simulink model "Three_Phase_Templates"  (R2021a)
settings: Solver=VariableStepAuto  StartTime=0.0  StopTime=10.0  RelTol=1e-3
libraries: fl_lib x35, nesl_utility x22, ee_lib x7, spsFourierLib x3, simulink_extras x1
settings Model: Creator=bemen  LastModifiedBy=bemen

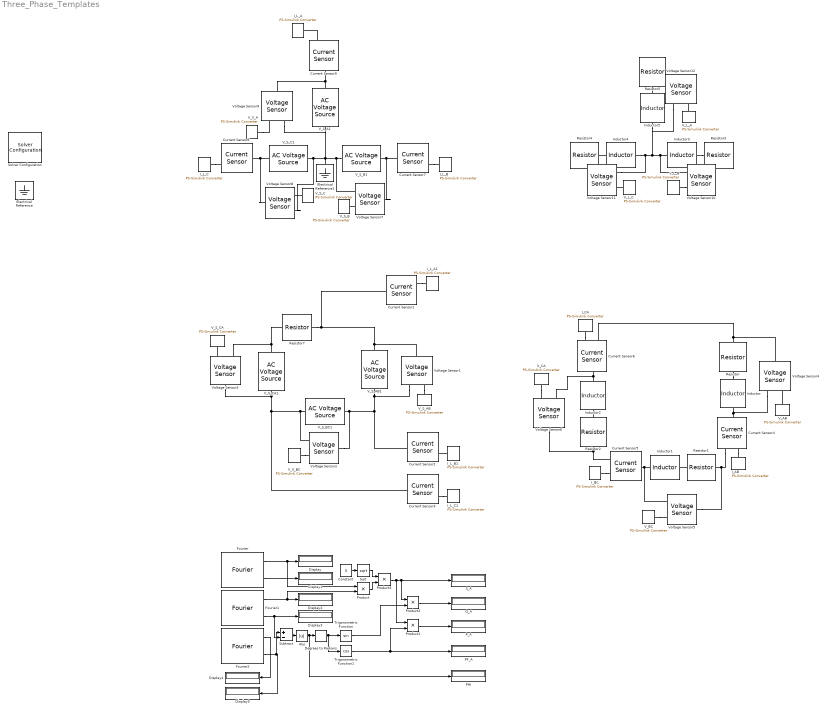
== system Three_Phase_Templates ==
  Abs : Abs
  Constant : Constant  Value=3
  Current Sensor{1..9} (9 alike) : fl_lib/Electrical/Electrical Sensors/Current Sensor
  Degrees to Radians : simulink_extras/Transformations/Degrees to Radians
  Display{,1..5} (6 alike) : Display
  Electrical Reference : fl_lib/Electrical/Electrical Elements/Electrical Reference
  Electrical Reference1 : fl_lib/Electrical/Electrical Elements/Electrical Reference
  Fourier : spsFourierLib/Fourier  Freq=60  n=1  InInit=[0, 0]  Ts=0
      settings: SourceProductBaseCode=PS
  Fourier1 : spsFourierLib/Fourier  Freq=60  n=1  InInit=[0, 0]  Ts=0
      settings: SourceProductBaseCode=PS
  Fourier2 : spsFourierLib/Fourier  Freq=60  n=1  InInit=[0, 0]  Ts=0
      settings: SourceProductBaseCode=PS
  I_AB : nesl_utility/PS-Simulink Converter  PhysicalDomain=network_engine_domain  SubClassName=ps_output  LeftPortType=input  RightPortType=output  PseudoPeriodic=off  Frequencies=[]  Unit=inherit  AffineConversion=off
      settings: SourceProductBaseCode=PW,SS
  I_BC : nesl_utility/PS-Simulink Converter  PhysicalDomain=network_engine_domain  SubClassName=ps_output  LeftPortType=input  RightPortType=output  PseudoPeriodic=off  Frequencies=[]  Unit=inherit  AffineConversion=off
      settings: SourceProductBaseCode=PW,SS
  I_CA : nesl_utility/PS-Simulink Converter  PhysicalDomain=network_engine_domain  SubClassName=ps_output  LeftPortType=input  RightPortType=output  PseudoPeriodic=off  Frequencies=[]  Unit=inherit  AffineConversion=off
      settings: SourceProductBaseCode=PW,SS
  I_L_A : nesl_utility/PS-Simulink Converter  PhysicalDomain=network_engine_domain  SubClassName=ps_output  LeftPortType=input  RightPortType=output  PseudoPeriodic=off  Frequencies=[]  Unit=inherit  AffineConversion=off
      settings: SourceProductBaseCode=PW,SS
  I_L_A1 : nesl_utility/PS-Simulink Converter  PhysicalDomain=network_engine_domain  SubClassName=ps_output  LeftPortType=input  RightPortType=output  PseudoPeriodic=off  Frequencies=[]  Unit=inherit  AffineConversion=off
      settings: SourceProductBaseCode=PW,SS
  I_L_B : nesl_utility/PS-Simulink Converter  PhysicalDomain=network_engine_domain  SubClassName=ps_output  LeftPortType=input  RightPortType=output  PseudoPeriodic=off  Frequencies=[]  Unit=inherit  AffineConversion=off
      settings: SourceProductBaseCode=PW,SS
  I_L_B1 : nesl_utility/PS-Simulink Converter  PhysicalDomain=network_engine_domain  SubClassName=ps_output  LeftPortType=input  RightPortType=output  PseudoPeriodic=off  Frequencies=[]  Unit=inherit  AffineConversion=off
      settings: SourceProductBaseCode=PW,SS
  I_L_C : nesl_utility/PS-Simulink Converter  PhysicalDomain=network_engine_domain  SubClassName=ps_output  LeftPortType=input  RightPortType=output  PseudoPeriodic=off  Frequencies=[]  Unit=inherit  AffineConversion=off
      settings: SourceProductBaseCode=PW,SS
  I_L_C1 : nesl_utility/PS-Simulink Converter  PhysicalDomain=network_engine_domain  SubClassName=ps_output  LeftPortType=input  RightPortType=output  PseudoPeriodic=off  Frequencies=[]  Unit=inherit  AffineConversion=off
      settings: SourceProductBaseCode=PW,SS
  Inductor{,1..5} (6 alike) : fl_lib/Electrical/Electrical Elements/Inductor  l=13.26291192 mH  r=0 Ohm  g=1e-9 1/Ohm  i_specify=off  i_priority=None  i=0 A  i_nominal_specify=off  i_nominal_unit=A  i_nominal_value=1  v_specify=off  v_priority=None  v=0 V  v_nominal_specify=off  v_nominal_unit=V  v_nominal_value=1  i_L_specify=off  i_L_priority=High  i_L=0 A  i_L_nominal_specify=off  i_L_nominal_unit=A  i_L_nominal_value=1
  PF_A : Display
  PHI : Display
  P_A : Display
  Product{,1..3} (4 alike) : Product
  Q_A : Display
  Resistor : ee_lib/Passive/Resistor  R=5 Ohm  R_tol=5  enable_R_tol=0  tol_distribution=1  nSigma=4  enable_operating_limits=0  operating_limit_action=2  max_working_voltage=100 V  power_rating=1 W  enable_faults=0  fault_action=1  R_faulted=inf Ohm  enable_temporal_fault=0  t_fault=1 s  enable_behavioral_fault=0  max_permissible_current=1 A  t_fail_on_current=1 s  noise_mode=0  sample_time=1e-3 s  repeatability=1  auto_seed=19903842  user_seed=0  Tdevice=25 degC  alpha=3.93e-3 1/K  Tmeas=25 degC  thermal_mass=100 J/K  power_derating_T1=70 degC  power_derating_T2=155 degC  operating_temperature_range_vec=[-50, 150] degC  temperature_specify=off  temperature_priority=High  temperature=298.15 K  temperature_nominal_specify=off  temperature_nominal_unit=K  temperature_nominal_value=1
  Resistor1 : ee_lib/Passive/Resistor  R=5 Ohm  R_tol=5  enable_R_tol=0  tol_distribution=1  nSigma=4  enable_operating_limits=0  operating_limit_action=2  max_working_voltage=100 V  power_rating=1 W  enable_faults=0  fault_action=1  R_faulted=inf Ohm  enable_temporal_fault=0  t_fault=1 s  enable_behavioral_fault=0  max_permissible_current=1 A  t_fail_on_current=1 s  noise_mode=0  sample_time=1e-3 s  repeatability=1  auto_seed=3510290603  user_seed=0  Tdevice=25 degC  alpha=3.93e-3 1/K  Tmeas=25 degC  thermal_mass=100 J/K  power_derating_T1=70 degC  power_derating_T2=155 degC  operating_temperature_range_vec=[-50, 150] degC  temperature_specify=off  temperature_priority=High  temperature=298.15 K  temperature_nominal_specify=off  temperature_nominal_unit=K  temperature_nominal_value=1
  Resistor2 : ee_lib/Passive/Resistor  R=5 Ohm  R_tol=5  enable_R_tol=0  tol_distribution=1  nSigma=4  enable_operating_limits=0  operating_limit_action=2  max_working_voltage=100 V  power_rating=1 W  enable_faults=0  fault_action=1  R_faulted=inf Ohm  enable_temporal_fault=0  t_fault=1 s  enable_behavioral_fault=0  max_permissible_current=1 A  t_fail_on_current=1 s  noise_mode=0  sample_time=1e-3 s  repeatability=1  auto_seed=3731015349  user_seed=0  Tdevice=25 degC  alpha=3.93e-3 1/K  Tmeas=25 degC  thermal_mass=100 J/K  power_derating_T1=70 degC  power_derating_T2=155 degC  operating_temperature_range_vec=[-50, 150] degC  temperature_specify=off  temperature_priority=High  temperature=298.15 K  temperature_nominal_specify=off  temperature_nominal_unit=K  temperature_nominal_value=1
  Resistor3 : ee_lib/Passive/Resistor  R=5 Ohm  R_tol=5  enable_R_tol=0  tol_distribution=1  nSigma=4  enable_operating_limits=0  operating_limit_action=2  max_working_voltage=100 V  power_rating=1 W  enable_faults=0  fault_action=1  R_faulted=inf Ohm  enable_temporal_fault=0  t_fault=1 s  enable_behavioral_fault=0  max_permissible_current=1 A  t_fail_on_current=1 s  noise_mode=0  sample_time=1e-3 s  repeatability=1  auto_seed=362649195  user_seed=0  Tdevice=25 degC  alpha=3.93e-3 1/K  Tmeas=25 degC  thermal_mass=100 J/K  power_derating_T1=70 degC  power_derating_T2=155 degC  operating_temperature_range_vec=[-50, 150] degC  temperature_specify=off  temperature_priority=High  temperature=298.15 K  temperature_nominal_specify=off  temperature_nominal_unit=K  temperature_nominal_value=1
  Resistor4 : ee_lib/Passive/Resistor  R=5 Ohm  R_tol=5  enable_R_tol=0  tol_distribution=1  nSigma=4  enable_operating_limits=0  operating_limit_action=2  max_working_voltage=100 V  power_rating=1 W  enable_faults=0  fault_action=1  R_faulted=inf Ohm  enable_temporal_fault=0  t_fault=1 s  enable_behavioral_fault=0  max_permissible_current=1 A  t_fail_on_current=1 s  noise_mode=0  sample_time=1e-3 s  repeatability=1  auto_seed=1717053403  user_seed=0  Tdevice=25 degC  alpha=3.93e-3 1/K  Tmeas=25 degC  thermal_mass=100 J/K  power_derating_T1=70 degC  power_derating_T2=155 degC  operating_temperature_range_vec=[-50, 150] degC  temperature_specify=off  temperature_priority=High  temperature=298.15 K  temperature_nominal_specify=off  temperature_nominal_unit=K  temperature_nominal_value=1
  Resistor5 : ee_lib/Passive/Resistor  R=5 Ohm  R_tol=5  enable_R_tol=0  tol_distribution=1  nSigma=4  enable_operating_limits=0  operating_limit_action=2  max_working_voltage=100 V  power_rating=1 W  enable_faults=0  fault_action=1  R_faulted=inf Ohm  enable_temporal_fault=0  t_fault=1 s  enable_behavioral_fault=0  max_permissible_current=1 A  t_fail_on_current=1 s  noise_mode=0  sample_time=1e-3 s  repeatability=1  auto_seed=1116134882  user_seed=0  Tdevice=25 degC  alpha=3.93e-3 1/K  Tmeas=25 degC  thermal_mass=100 J/K  power_derating_T1=70 degC  power_derating_T2=155 degC  operating_temperature_range_vec=[-50, 150] degC  temperature_specify=off  temperature_priority=High  temperature=298.15 K  temperature_nominal_specify=off  temperature_nominal_unit=K  temperature_nominal_value=1
  Resistor7 : ee_lib/Passive/Resistor  R=0.000001 Ohm  R_tol=5  enable_R_tol=0  tol_distribution=1  nSigma=4  enable_operating_limits=0  operating_limit_action=2  max_working_voltage=100 V  power_rating=1 W  enable_faults=0  fault_action=1  R_faulted=inf Ohm  enable_temporal_fault=0  t_fault=1 s  enable_behavioral_fault=0  max_permissible_current=1 A  t_fail_on_current=1 s  noise_mode=0  sample_time=1e-3 s  repeatability=1  auto_seed=189689687  user_seed=0  Tdevice=25 degC  alpha=3.93e-3 1/K  Tmeas=25 degC  thermal_mass=100 J/K  power_derating_T1=70 degC  power_derating_T2=155 degC  operating_temperature_range_vec=[-50, 150] degC  temperature_specify=off  temperature_priority=High  temperature=298.15 K  temperature_nominal_specify=off  temperature_nominal_unit=K  temperature_nominal_value=1
  S_A : Display
  Solver Configuration : nesl_utility/Solver Configuration  PhysicalDomain=network_engine_domain  SubClassName=solver  LeftPortType=input  RightPortType=generic  Tones=[]  Harmonics=[]  SimulateNoise=off  Profile=off  UseLocalSampling=off  EnableSwitchedLinearOptims=on  FrequencyDomain=off  UseCCode=off  RelTol=0.001  AbsTol=1e-06  MinStep=1e-09  ToWorkspace=off  RevertToSquareIcSolve=off  NumHomotopyIterations=100  PhasorMode=off  PhasorModeNumHarmonics=1  DoDC=on  ResidualTolerance=1e-09  UseLocalSolver=off  LocalSolverChoice=NE_BACKWARD_EULER_ADVANCER  LocalSolverSampleTime=0.001  DoFixedCost=off  MaxNonlinIter=3  MaxModeIter=2  ComputeImpulses=off  ImpulseIterations=2  LinearAlgebra=auto  EquationFormulation=NE_TIME_EF  DelaysMemoryBudget=1024  AutomaticFiltering=on  FilteringTimeConstant=0.001  PartitionStorageMethod=AS_NEEDED  PartitionMemoryBudget=1024  PartitionMethod=ROBUST
      settings: SourceProductBaseCode=PW,SS
  Sqrt : Sqrt  SaturateOnIntegerOverflow=on
  Subtract : Sum  Inputs=+-
  Trigonometric Function : Trigonometry
  Trigonometric Function1 : Trigonometry  Operator=cos
  V_AB : nesl_utility/PS-Simulink Converter  PhysicalDomain=network_engine_domain  SubClassName=ps_output  LeftPortType=input  RightPortType=output  PseudoPeriodic=off  Frequencies=[]  Unit=inherit  AffineConversion=off
      settings: SourceProductBaseCode=PW,SS
  V_BC : nesl_utility/PS-Simulink Converter  PhysicalDomain=network_engine_domain  SubClassName=ps_output  LeftPortType=input  RightPortType=output  PseudoPeriodic=off  Frequencies=[]  Unit=inherit  AffineConversion=off
      settings: SourceProductBaseCode=PW,SS
  V_CA : nesl_utility/PS-Simulink Converter  PhysicalDomain=network_engine_domain  SubClassName=ps_output  LeftPortType=input  RightPortType=output  PseudoPeriodic=off  Frequencies=[]  Unit=inherit  AffineConversion=off
      settings: SourceProductBaseCode=PW,SS
  V_L_A : nesl_utility/PS-Simulink Converter  PhysicalDomain=network_engine_domain  SubClassName=ps_output  LeftPortType=input  RightPortType=output  PseudoPeriodic=off  Frequencies=[]  Unit=inherit  AffineConversion=off
      settings: SourceProductBaseCode=PW,SS
  V_L_B : nesl_utility/PS-Simulink Converter  PhysicalDomain=network_engine_domain  SubClassName=ps_output  LeftPortType=input  RightPortType=output  PseudoPeriodic=off  Frequencies=[]  Unit=inherit  AffineConversion=off
      settings: SourceProductBaseCode=PW,SS
  V_L_C : nesl_utility/PS-Simulink Converter  PhysicalDomain=network_engine_domain  SubClassName=ps_output  LeftPortType=input  RightPortType=output  PseudoPeriodic=off  Frequencies=[]  Unit=inherit  AffineConversion=off
      settings: SourceProductBaseCode=PW,SS
  V_S_A : nesl_utility/PS-Simulink Converter  PhysicalDomain=network_engine_domain  SubClassName=ps_output  LeftPortType=input  RightPortType=output  PseudoPeriodic=off  Frequencies=[]  Unit=inherit  AffineConversion=off
      settings: SourceProductBaseCode=PW,SS
  V_S_A1 : fl_lib/Electrical/Electrical Sources/AC Voltage Source  amp=120 V  shift=0 deg  frequency=60 Hz  omega=0 rad/s
  V_S_AB : nesl_utility/PS-Simulink Converter  PhysicalDomain=network_engine_domain  SubClassName=ps_output  LeftPortType=input  RightPortType=output  PseudoPeriodic=off  Frequencies=[]  Unit=inherit  AffineConversion=off
      settings: SourceProductBaseCode=PW,SS
  V_S_AB1 : fl_lib/Electrical/Electrical Sources/AC Voltage Source  amp=120 V  shift=0 deg  frequency=60 Hz  omega=0 rad/s
  V_S_B : nesl_utility/PS-Simulink Converter  PhysicalDomain=network_engine_domain  SubClassName=ps_output  LeftPortType=input  RightPortType=output  PseudoPeriodic=off  Frequencies=[]  Unit=inherit  AffineConversion=off
      settings: SourceProductBaseCode=PW,SS
  V_S_B1 : fl_lib/Electrical/Electrical Sources/AC Voltage Source  amp=120 V  shift=-120 deg  frequency=60 Hz  omega=0 rad/s
  V_S_BC : nesl_utility/PS-Simulink Converter  PhysicalDomain=network_engine_domain  SubClassName=ps_output  LeftPortType=input  RightPortType=output  PseudoPeriodic=off  Frequencies=[]  Unit=inherit  AffineConversion=off
      settings: SourceProductBaseCode=PW,SS
  V_S_BC1 : fl_lib/Electrical/Electrical Sources/AC Voltage Source  amp=120 V  shift=-120 deg  frequency=60 Hz  omega=0 rad/s
  V_S_C : nesl_utility/PS-Simulink Converter  PhysicalDomain=network_engine_domain  SubClassName=ps_output  LeftPortType=input  RightPortType=output  PseudoPeriodic=off  Frequencies=[]  Unit=inherit  AffineConversion=off
      settings: SourceProductBaseCode=PW,SS
  V_S_C1 : fl_lib/Electrical/Electrical Sources/AC Voltage Source  amp=120 V  shift=120 deg  frequency=60 Hz  omega=0 rad/s
  V_S_CA : nesl_utility/PS-Simulink Converter  PhysicalDomain=network_engine_domain  SubClassName=ps_output  LeftPortType=input  RightPortType=output  PseudoPeriodic=off  Frequencies=[]  Unit=inherit  AffineConversion=off
      settings: SourceProductBaseCode=PW,SS
  V_S_CA1 : fl_lib/Electrical/Electrical Sources/AC Voltage Source  amp=120 V  shift=120 deg  frequency=60 Hz  omega=0 rad/s
  Voltage Sensor{1..12} (12 alike) : fl_lib/Electrical/Electrical Sensors/Voltage Sensor
  wires:
  Fourier2/1 -> Display4/1
  Product3/1 -> Product1/1, Product2/1, S_A/1
  Product/1 -> Product3/2
  Fourier1/1 -> Product/2, Display2/1
  Abs/1 -> PHI/1, Degrees to Radians/1
  Product1/1 -> P_A/1
  Fourier/1 -> Product/1, Display/1
  Constant/1 -> Sqrt/1
  Sqrt/1 -> Product3/1
  Product2/1 -> Q_A/1
  Fourier/2 -> Display1/1
  Degrees to Radians/1 -> Trigonometric Function1/1, Trigonometric Function/1
  Trigonometric Function/1 -> Product2/2
  Trigonometric Function1/1 -> Product1/2, PF_A/1
  Fourier1/2 -> Subtract/2, Display3/1
  Fourier2/2 -> Subtract/1, Display5/1
  Subtract/1 -> Abs/1
  connections:
  V_S_AB1/RConn1 -- Voltage Sensor1/RConn2 -- Current Sensor2/LConn1 -- Voltage Sensor2/LConn1 -- V_S_BC1/LConn1
  V_S_BC1/RConn1 -- Voltage Sensor2/RConn2 -- Voltage Sensor3/LConn1 -- V_S_CA1/LConn1 -- Current Sensor3/LConn1
  Voltage Sensor3/RConn2 -- V_S_CA1/RConn1 -- Resistor7/LConn1
  Inductor/RConn1 -- Current Sensor4/LConn1 -- Voltage Sensor4/RConn2
  Resistor/RConn1 -- Inductor/LConn1
  Resistor1/RConn1 -- Inductor1/LConn1
  Resistor2/RConn1 -- Inductor2/LConn1
  Inductor2/RConn1 -- Voltage Sensor6/RConn2 -- Current Sensor6/LConn1
  Inductor1/RConn1 -- Voltage Sensor5/RConn2 -- Current Sensor5/LConn1
  Current Sensor6/RConn2 -- Voltage Sensor4/LConn1 -- Resistor/LConn1
  Resistor2/LConn1 -- Voltage Sensor6/LConn1 -- Current Sensor5/RConn2
  Current Sensor4/RConn2 -- Voltage Sensor5/LConn1 -- Resistor1/LConn1
  Current Sensor4/RConn1 -- I_AB/LConn1
  V_AB/LConn1 -- Voltage Sensor4/RConn1
  V_BC/LConn1 -- Voltage Sensor5/RConn1
  I_BC/LConn1 -- Current Sensor5/RConn1
  V_CA/LConn1 -- Voltage Sensor6/RConn1
  I_CA/LConn1 -- Current Sensor6/RConn1
  Voltage Sensor7/LConn1 -- Current Sensor7/LConn1 -- V_S_B1/LConn1
  V_S_C1/LConn1 -- Voltage Sensor8/LConn1 -- Current Sensor8/LConn1
  V_S_C1/RConn1 -- Voltage Sensor8/RConn2 -- Voltage Sensor9/RConn2 -- V_S_A1/RConn1 -- Electrical Reference1/LConn1 -- Voltage Sensor7/RConn2 -- V_S_B1/RConn1
  V_S_A1/LConn1 -- Voltage Sensor9/LConn1 -- Current Sensor9/LConn1
  Inductor3/LConn1 -- Resistor3/RConn1
  Inductor4/LConn1 -- Resistor4/RConn1
  Inductor5/LConn1 -- Resistor5/RConn1
  Inductor4/RConn1 -- Voltage Sensor11/RConn2 -- Voltage Sensor12/RConn2 -- Inductor5/RConn1 -- Voltage Sensor10/RConn2 -- Inductor3/RConn1
  V_L_B/LConn1 -- Voltage Sensor10/RConn1
  V_L_C/LConn1 -- Voltage Sensor11/RConn1
  V_L_A/LConn1 -- Voltage Sensor12/RConn1
  V_S_B/LConn1 -- Voltage Sensor7/RConn1
  V_S_C/LConn1 -- Voltage Sensor8/RConn1
  V_S_A/LConn1 -- Voltage Sensor9/RConn1
  Current Sensor7/RConn1 -- I_L_B/LConn1
  I_L_C/LConn1 -- Current Sensor8/RConn1
  Current Sensor9/RConn1 -- I_L_A/LConn1
  Voltage Sensor1/RConn1 -- V_S_AB/LConn1
  I_L_B1/LConn1 -- Current Sensor2/RConn1
  Current Sensor3/RConn1 -- I_L_C1/LConn1
  V_S_BC/LConn1 -- Voltage Sensor2/RConn1
  Voltage Sensor3/RConn1 -- V_S_CA/LConn1
  Current Sensor1/RConn1 -- I_L_A1/LConn1
  Current Sensor1/LConn1 -- V_S_AB1/LConn1 -- Voltage Sensor1/LConn1 -- Resistor7/RConn1
